simulink model "serial_test"  (R2020b)
settings: Solver=ode1be  StartTime=0.0  StopTime=inf  RelTol=1e-3
undefined symbols (not defined in the file or in its folder): LF, serial
libraries: instrumentlib x3, etargetslib x2
settings Model: EnablePacing=on  Creator=akern  LastModifiedBy=akern

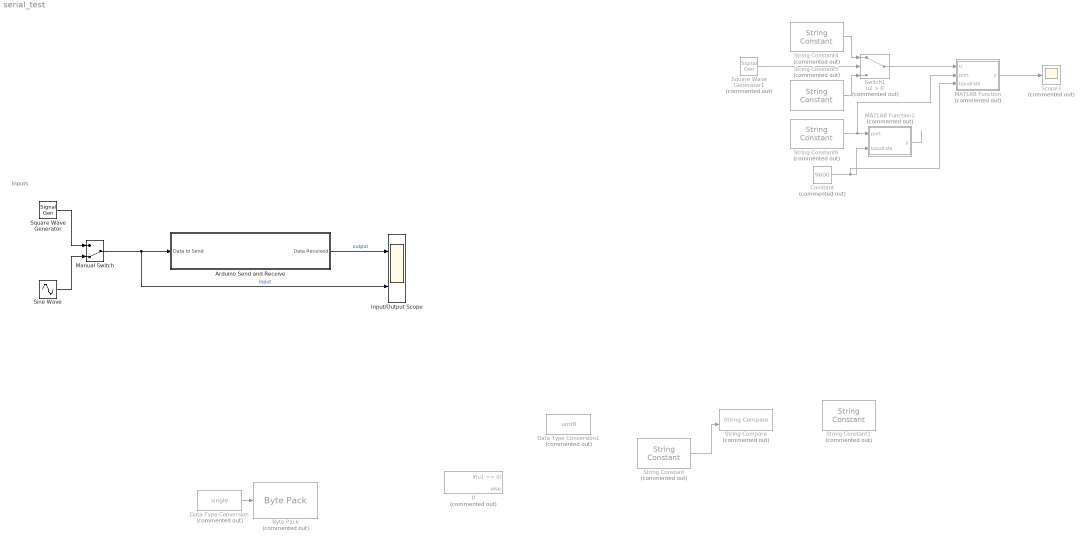
== system serial_test ==
  note: Inputs
  Arduino Send and Receive : Subsystem
  Byte Pack : etargetslib/Byte Pack  Commented=on  datatypes={'single'}  byteAlign=4
  Constant : Constant  Commented=on  Value=9600
  Data Type Conversion : DataTypeConversion  Commented=on  OutDataTypeStr=single
  Data Type Conversion1 : DataTypeConversion  Commented=on  OutDataTypeStr=uint8
  If : If  Commented=on  IfExpression=u1 == 0
  Input/Output Scope : Scope  NumInputPorts=2
  MATLAB Function : MATLAB Function  Commented=on  TreatAsAtomicUnit=on
  MATLAB Function1 : MATLAB Function  Commented=on  TreatAsAtomicUnit=on
  Manual Switch : ManualSwitch  CurrentSetting=0
  Scope3 : Scope  Commented=on
  Sine Wave : Sin  SampleTime=0
  Square Wave Generator : SignalGenerator  WaveForm=square  Units=rad/sec
  Square Wave Generator1 : SignalGenerator  Commented=on  WaveForm=square  Units=rad/sec
  String Compare : StringCompare  Commented=on
  String Constant : StringConstant  Commented=on  String="\"ON\""
  String Constant1 : StringConstant  Commented=on  String="\"OFF\""
  String Constant4 : StringConstant  Commented=on  String="\"ON\""
  String Constant5 : StringConstant  Commented=on  String="\"OFF\""
  String Constant6 : StringConstant  Commented=on  String="\"COM3\""
  Switch1 : Switch  Commented=on  Criteria=u2 > Threshold
  wires:
  Manual Switch/1 -> Input/Output Scope/2, Arduino Send and Receive/1(Data to Send)  "input"
  Data Type Conversion/1 -> Byte Pack/1
  String Constant5/1 -> Switch1/3
  String Constant4/1 -> Switch1/1
  Switch1/1 -> MATLAB Function/1(u)
  Square Wave Generator1/1 -> Switch1/2
  MATLAB Function/1(y) -> Scope3/1
  MATLAB Function1/1(y) -> ?
  String Constant6/1 -> MATLAB Function/2(port), MATLAB Function1/1(port)
  Constant/1 -> MATLAB Function/3(baudrate), MATLAB Function1/2(baudrate)
  String Constant/1 -> String Compare/2
  Arduino Send and Receive/1(Data Received) -> Input/Output Scope/1  "output"
  Square Wave Generator/1 -> Manual Switch/1
  Sine Wave/1 -> Manual Switch/2

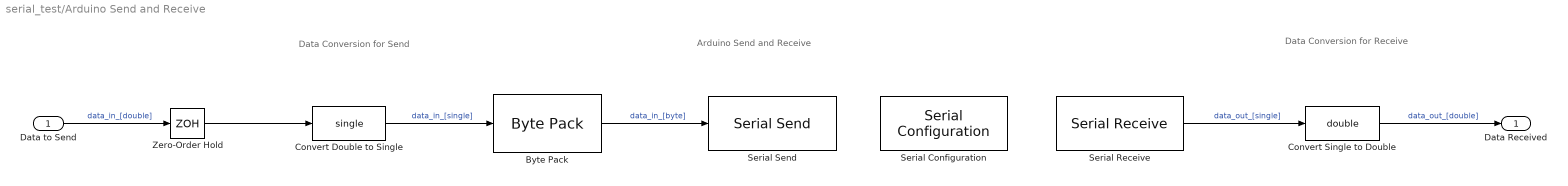
== system serial_test/Arduino Send and Receive ==
  note: Arduino Send and Receive
  note: Data Conversion
      | for Receive
  note: Data Conversion for Send
  Data to Send : Inport
  Byte Pack : etargetslib/Byte Pack  datatypes={'single'}  byteAlign=4
  Convert Double to Single : DataTypeConversion  OutDataTypeStr=single
  Convert Single to Double : DataTypeConversion  OutDataTypeStr=double
  Serial Configuration : instrumentlib/Serial Configuration  Priority=-200000  ComPortMenu=COM3  ComPort=COM3  ObjConstructor=serial('COM3');  BaudRate=115200  DataBits=8  Parity=none  StopBits=1  FlowControl=none  Timeout=10  ByteOrder=LittleEndian
  Serial Receive : instrumentlib/Serial Receive  ComPortMenu=COM3  ComPort=COM3  ObjConstructor=serial('COM3');  Header=A  Terminator=LF ('\n')  DataSize=[1 1]  DataType=single  EnableBlockingMode=on  ActionDataUnavailable=Output last received value  CustomValue=0  SampleTime=0.05
  Serial Send : instrumentlib/Serial Send  ComPortMenu=COM3  ComPort=COM3  ObjConstructor=serial('COM3');  Terminator=<none>  EnableBlockingMode=on
  Zero-Order Hold : ZeroOrderHold  SampleTime=0.05
  Data Received : Outport
  wires:
  Byte Pack/1 -> Serial Send/1  "data_in_[byte]"
  Convert Double to Single/1 -> Byte Pack/1  "data_in_[single]"
  Convert Single to Double/1 -> Data Received/1  "data_out_[double]"
  Zero-Order Hold/1 -> Convert Double to Single/1
  Serial Receive/1 -> Convert Single to Double/1  "data_out_[single]"
  Data to Send/1 -> Zero-Order Hold/1  "data_in_[double]"

== matlab function serial_test/MATLAB Function ==
  data: u input; y output; port input; baudrate input
function y = fcn(u, port, baudrate)
    arduino = serialport(port, baudrate);
    writeline(arduino, u);
y = u;

== matlab function serial_test/MATLAB Function1 ==
  data: port input; y output; baudrate input
function y = fcn(port, baudrate)
    serialport(port, baudrate);
y = u;
